simulink model "watercontentsimulaion"  (R2021b)
settings: Solver=FixedStepAuto  StartTime=0.0  StopTime=3000000  FixedStep=1  RelTol=1e-3
libraries: vrlib x2
settings Model: Creator=Nicolas Sicard  LastModifiedBy=Nicolas Sicard

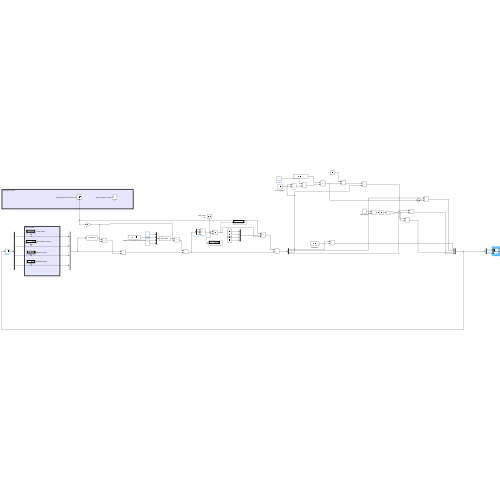
[thumbnail: Simulink's stored preview of the top-level diagram]
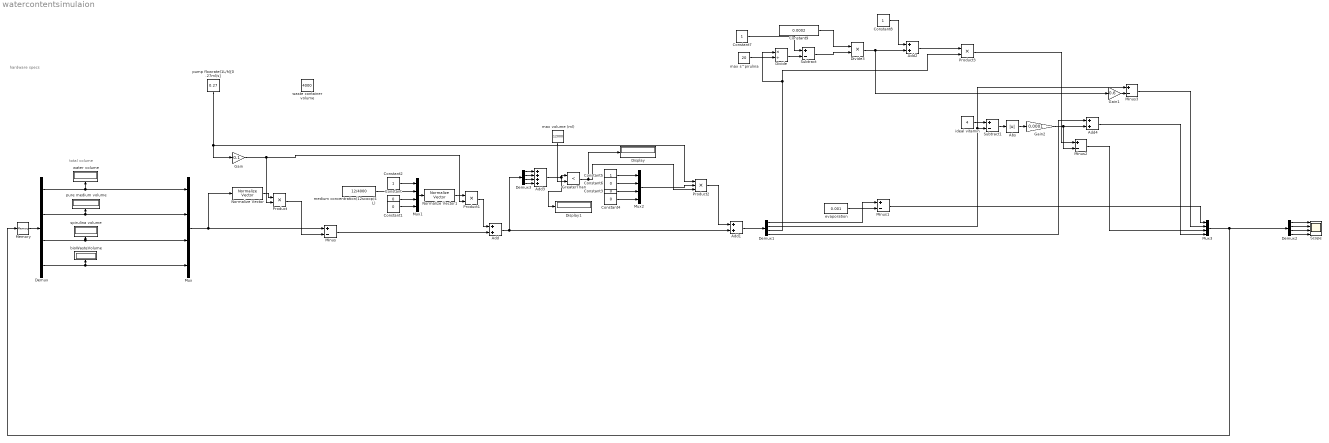
== system watercontentsimulaion ==
  note: total volume
  note: hardware specs
  Abs : Abs
  Add{,1..2,4} (4 alike) : Sum
  Add3 : Sum  Inputs=++++
  Constant{,1,3..4,6} (5 alike) : Constant  Value=0
  Constant{2,5,7..8} (4 alike) : Constant
  Constant9 : Constant  Value=0.0002
  Demux{,1..3} (4 alike) : Demux
  Display : Display
  Display1 : Display
  Divide : Product  Inputs=*/
  Divide3 : Product  Inputs=**
  Gain : Gain  Gain=0.1
  Gain1 : Gain  Gain=0.6
  Gain2 : Gain  Gain=0.0001
  GreaterThan : RelationalOperator  Operator=<  OutDataTypeStr=boolean  RndMeth=Simplest
  Memory : Memory  InitialCondition=[12000 2 2 0]  LinearizeAsDelay=on
  Minus{,1..3} (4 alike) : Sum  Inputs=+-
  Mux{,1..3} (4 alike) : Mux
  Normalize Vector : vrlib/Utilities/Normalize Vector  maxzero=0
  Normalize Vector1 : vrlib/Utilities/Normalize Vector  maxzero=0
  Product : Product
  Product1 : Product
  Product2 : Product  Inputs=3
  Product3 : Product
  Scope : Scope  NumInputPorts=4
  Subtract : Sum  Inputs=+-
  Subtract1 : Sum  Inputs=+-
  bioWasteVolume : Display
  evaporation : Constant  Value=0.001
  ideal vitamin : Constant  Value=4
  "max s^pirulina " : Constant  Value=20
  max volume (ml) : Constant  Value=12000
  medium concentration(12scoop/4L) : Constant  Value=12/4000
  pump flowrate(1L/h)[0.27ml/s] : Constant  Value=0.27
  pure medium volume : Display
  spirulina volume : Display
  waste container volume : Constant  Value=4000
  water volume : Display
  wires:
  Mux/1 -> Minus/1, Normalize Vector/1
  Demux/1 -> Mux/1, water volume/1
  Demux/2 -> Mux/2, pure medium volume/1
  Demux/3 -> Mux/3, spirulina volume/1
  Demux/4 -> Mux/4, bioWasteVolume/1
  Memory/1 -> Demux/1
  Normalize Vector/1 -> Product/1
  pump flowrate(1L/h)[0.27ml/s]/1 -> Gain/1, Product2/1
  Minus/1 -> Add/2
  Product/1 -> Minus/2
  Constant1/1 -> Mux1/4
  Constant/1 -> Mux1/3
  medium concentration(12scoop/4L)/1 -> Mux1/2
  Constant2/1 -> Mux1/1
  Normalize Vector1/1 -> Product1/1
  Mux1/1 -> Normalize Vector1/1
  Add/1 -> Add1/2, Demux3/1
  Product1/1 -> Add/1
  Add3/1 -> GreaterThan/1, Display1/1
  max volume (ml)/1 -> GreaterThan/2
  Constant3/1 -> Mux2/3
  Constant4/1 -> Mux2/4
  Constant6/1 -> Mux2/2
  Constant5/1 -> Mux2/1
  Mux2/1 -> Product2/2
  Product2/1 -> Add1/1
  Demux1/3 -> Divide/1, Product3/2
  GreaterThan/1 -> Display/1, Product2/3
  Mux3/1 -> Memory/1, Demux2/1
  Add1/1 -> Demux1/1
  Demux1/1 -> Minus1/1
  Demux1/4 -> Add4/1
  Constant8/1 -> Add2/1
  Constant9/1 -> Divide3/1
  Add2/1 -> Product3/1
  "max s^pirulina "/1 -> Divide/2
  Divide/1 -> Subtract/2
  Divide3/1 -> Gain1/1, Add2/2
  Product3/1 -> Minus2/1
  Demux2/1 -> Scope/1
  Demux2/2 -> Scope/2
  Demux2/3 -> Scope/3
  Demux2/4 -> Scope/4
  Constant7/1 -> Subtract/1
  Subtract/1 -> Divide3/2
  Minus1/1 -> Mux3/1
  evaporation/1 -> Minus1/2
  Demux1/2 -> Subtract1/2, Minus3/1
  Gain/1 -> Product1/2, Product/2
  Demux3/1 -> Add3/1
  Demux3/2 -> Add3/2
  Demux3/3 -> Add3/3
  Demux3/4 -> Add3/4
  ideal vitamin/1 -> Subtract1/1
  Subtract1/1 -> Abs/1
  Gain2/1 -> Minus2/2, Add4/2
  Add4/1 -> Mux3/4
  Minus2/1 -> Mux3/3
  Minus3/1 -> Mux3/2
  Abs/1 -> Gain2/1
  Gain1/1 -> Minus3/2
